simulink model "simulink_model"  (R2022b)
settings: Solver=FixedStepAuto  StartTime=0.0  StopTime=max_time  FixedStep=dt  RelTol=1e-3
undefined symbols (not defined in the file): dampCoeff, delay, DiscIntNeverNeededParam, dt, final_target_ang, Inertia, Kd_feedback, Kd_forward, Kp_feedback, Kp_forward, mvt_start_time, pert_amp, pert_end_time, pert_start_time
settings Model: Creator=Marcel  LastModifiedBy=Marcel

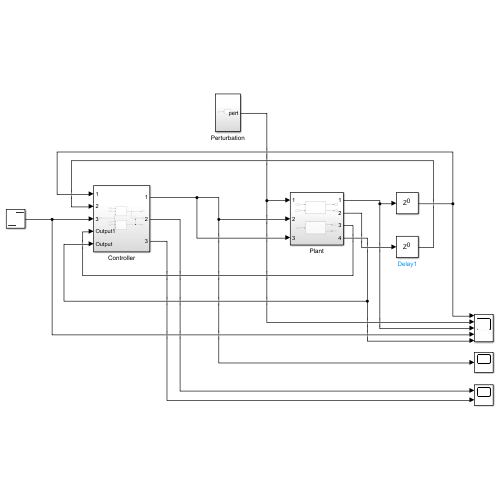
[thumbnail: Simulink's stored preview of the top-level diagram]
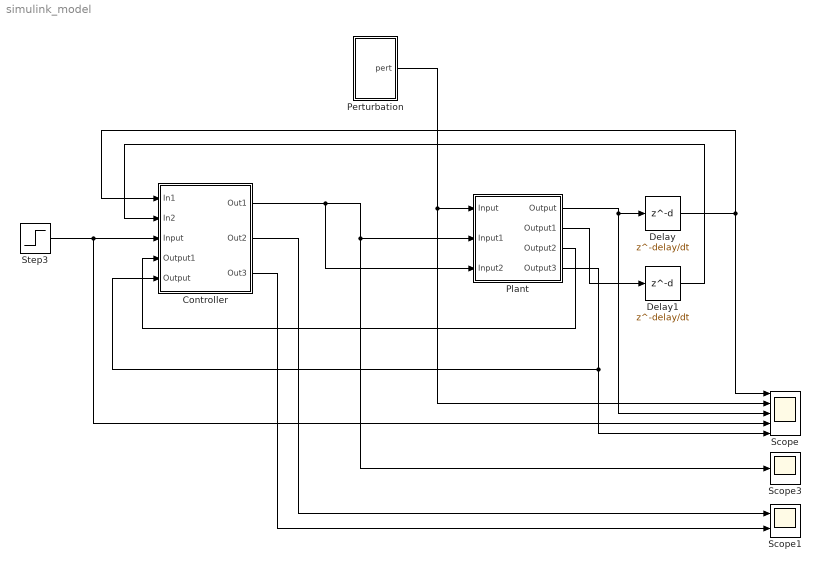
== system simulink_model ==
  Controller : Subsystem
  Delay : Delay  DelayLength=delay/dt
  Delay1 : Delay  DelayLength=delay/dt
  Perturbation : Subsystem
  Plant : Subsystem
  Scope : Scope  NumInputPorts=5
  Scope1 : Scope  NumInputPorts=2
  Scope3 : Scope
  Step3 : Step  Time=mvt_start_time  After=final_target_ang  SampleTime=0
  wires:
  Delay/1 -> Controller/1(In1), Scope/1
  Step3/1 -> Scope/4, Controller/3(Input)
  Perturbation/1(pert) -> Scope/2, Plant/1(Input)
  Controller/1(Out1) -> Scope3/1, Plant/2(Input1), Plant/3(Input2)
  Delay1/1 -> Controller/2(In2)
  Controller/2(Out2) -> Scope1/1
  Controller/3(Out3) -> Scope1/2
  Plant/4(Output3) -> Controller/5(Output), Scope/5
  Plant/1(Output) -> Scope/3, Delay/1
  Plant/2(Output1) -> Delay1/1
  Plant/3(Output2) -> Controller/4(Output1)

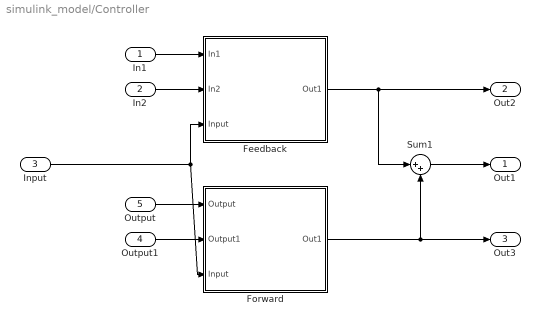
== system simulink_model/Controller ==
  In1 : Inport
  In2 : Inport  Port=2
  Input : Inport  Port=3
  Output1 : Inport  Port=4
  Output : Inport  Port=5
  Feedback : Subsystem
  Forward : Subsystem
  Sum1 : Sum  Inputs=|++
  Out1 : Outport
  Out2 : Outport  Port=2
  Out3 : Outport  Port=3
  wires:
  Forward/1(Out1) -> Out3/1, Sum1/2
  Feedback/1(Out1) -> Out2/1, Sum1/1
  In2/1 -> Feedback/2(In2)
  Sum1/1 -> Out1/1
  Output1/1 -> Forward/2(Output1)
  Output/1 -> Forward/1(Output)
  Input/1 -> Feedback/3(Input), Forward/3(Input)
  In1/1 -> Feedback/1(In1)

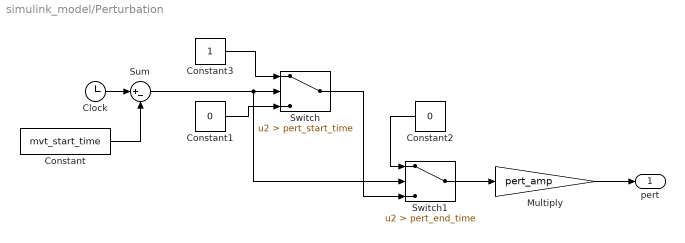
== system simulink_model/Perturbation ==
  Clock : Clock
  Constant : Constant  Value=mvt_start_time
  Constant1 : Constant  Value=0
  Constant2 : Constant  Value=0
  Constant3 : Constant
  Multiply : Gain  Gain=pert_amp
  Sum : Sum  Inputs=|+-
  Switch : Switch  Criteria=u2 > Threshold  Threshold=pert_start_time  SaturateOnIntegerOverflow=off  InputSameDT=off
  Switch1 : Switch  Criteria=u2 > Threshold  Threshold=pert_end_time  SaturateOnIntegerOverflow=off  InputSameDT=off
  pert : Outport
  wires:
  Switch1/1 -> Multiply/1
  Multiply/1 -> pert/1
  Clock/1 -> Sum/1
  Sum/1 -> Switch/2, Switch1/2
  Constant/1 -> Sum/2
  Switch/1 -> Switch1/3
  Constant3/1 -> Switch/1
  Constant1/1 -> Switch/3
  Constant2/1 -> Switch1/1

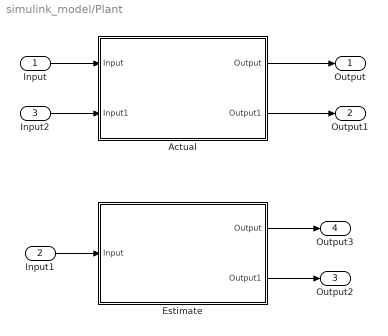
== system simulink_model/Plant ==
  Input : Inport
  Input1 : Inport  Port=2
  Input2 : Inport  Port=3
  Actual : Subsystem
  Estimate : Subsystem
  Output : Outport
  Output1 : Outport  Port=2
  Output2 : Outport  Port=3
  Output3 : Outport  Port=4
  wires:
  Input1/1 -> Estimate/1(Input)
  Actual/2(Output1) -> Output1/1
  Input2/1 -> Actual/2(Input1)
  Estimate/1(Output) -> Output3/1
  Estimate/2(Output1) -> Output2/1
  Actual/1(Output) -> Output/1
  Input/1 -> Actual/1(Input)

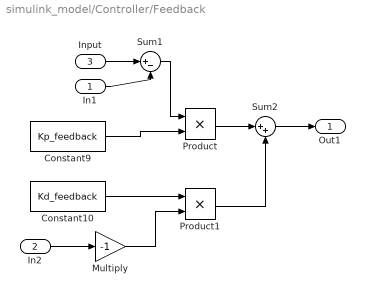
== system simulink_model/Controller/Feedback ==
  In1 : Inport
  In2 : Inport  Port=2
  Input : Inport  Port=3
  Constant10 : Constant  Value=Kd_feedback
  Constant9 : Constant  Value=Kp_feedback
  Multiply : Gain  Gain=-1
  Product : Product
  Product1 : Product
  Sum1 : Sum  Inputs=|+-
  Sum2 : Sum  Inputs=|++
  Out1 : Outport
  wires:
  Product1/1 -> Sum2/2
  In2/1 -> Multiply/1
  Sum1/1 -> Product/1
  Constant10/1 -> Product1/1
  Product/1 -> Sum2/1
  Constant9/1 -> Product/2
  In1/1 -> Sum1/2
  Sum2/1 -> Out1/1
  Input/1 -> Sum1/1
  Multiply/1 -> Product1/2

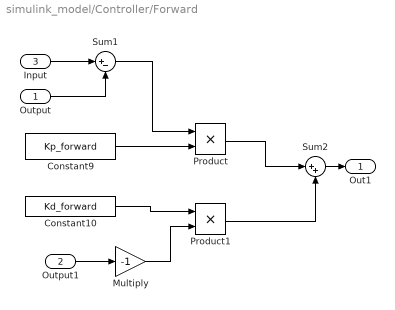
== system simulink_model/Controller/Forward ==
  Output : Inport
  Output1 : Inport  Port=2
  Input : Inport  Port=3
  Constant10 : Constant  Value=Kd_forward
  Constant9 : Constant  Value=Kp_forward
  Multiply : Gain  Gain=-1
  Product : Product
  Product1 : Product
  Sum1 : Sum  Inputs=|+-
  Sum2 : Sum  Inputs=|++
  Out1 : Outport
  wires:
  Product1/1 -> Sum2/2
  Output1/1 -> Multiply/1
  Sum1/1 -> Product/1
  Constant10/1 -> Product1/1
  Product/1 -> Sum2/1
  Constant9/1 -> Product/2
  Input/1 -> Sum1/1
  Output/1 -> Sum1/2
  Sum2/1 -> Out1/1
  Multiply/1 -> Product1/2

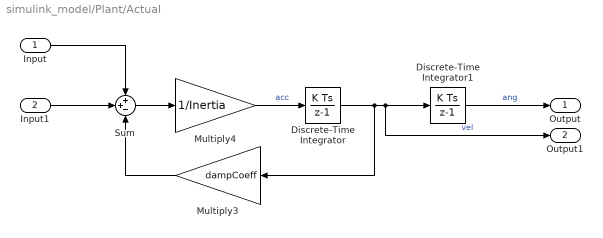
== system simulink_model/Plant/Actual ==
  Input : Inport
  Input1 : Inport  Port=2
  Discrete-Time Integrator : DiscreteIntegrator  SampleTime=-1  ICPrevOutput=DiscIntNeverNeededParam  ICPrevScaledInput=DiscIntNeverNeededParam
  Discrete-Time Integrator1 : DiscreteIntegrator  SampleTime=-1  ICPrevOutput=DiscIntNeverNeededParam  ICPrevScaledInput=DiscIntNeverNeededParam
  Multiply3 : Gain  Gain=dampCoeff
  Multiply4 : Gain  Gain=1/Inertia
  Sum : Sum  Inputs=++-
  Output : Outport
  Output1 : Outport  Port=2
  wires:
  Multiply4/1 -> Discrete-Time Integrator/1  "acc"
  Discrete-Time Integrator1/1 -> Output/1  "ang"
  Sum/1 -> Multiply4/1
  Discrete-Time Integrator/1 -> Output1/1, Discrete-Time Integrator1/1, Multiply3/1  "vel"
  Input/1 -> Sum/1
  Input1/1 -> Sum/2
  Multiply3/1 -> Sum/3

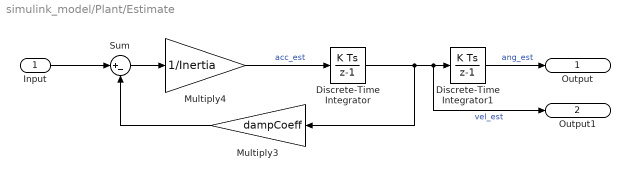
== system simulink_model/Plant/Estimate ==
  Input : Inport
  Discrete-Time Integrator : DiscreteIntegrator  SampleTime=-1  ICPrevOutput=DiscIntNeverNeededParam  ICPrevScaledInput=DiscIntNeverNeededParam
  Discrete-Time Integrator1 : DiscreteIntegrator  SampleTime=-1  ICPrevOutput=DiscIntNeverNeededParam  ICPrevScaledInput=DiscIntNeverNeededParam
  Multiply3 : Gain  Gain=dampCoeff
  Multiply4 : Gain  Gain=1/Inertia
  Sum : Sum  Inputs=|+-
  Output : Outport
  Output1 : Outport  Port=2
  wires:
  Input/1 -> Sum/1
  Multiply3/1 -> Sum/2
  Sum/1 -> Multiply4/1
  Multiply4/1 -> Discrete-Time Integrator/1  "acc_est"
  Discrete-Time Integrator/1 -> Discrete-Time Integrator1/1, Output1/1, Multiply3/1  "vel_est"
  Discrete-Time Integrator1/1 -> Output/1  "ang_est"
